simulink model "MCC"  (Simulink 9.0)
settings: Solver=ode15s  StartTime=0.0  StopTime=0.2  RelTol=1e-3
InitFcn:
  | MCC_constants
StartFcn:
  | MCC_constants
values from neighbouring files (symbols this model uses):
  b = 8.5E-3    (= 0.0085)    [TD2_config.m]
  J = 0.28    [TD2_config.m]
  K = 0.5093    [TD2_config.m]
  L = 1.6E-3    (= 0.0016)    [TD2_config.m]
  R = 0.13    [TD2_config.m]
settings Model: Creator=TABLE 6  LastModifiedBy=TABLE 6
settings DataIOCC: SaveFormat=Dataset
settings OptimizationCC: LifeSpan=auto
settings DebuggingCC: UnderspecifiedInitializationDetection=Simplified  MergeDetectMultiDrivingBlocksExec=error  SFUnexpectedBacktrackingDiag=error  SFNoUnconditionalDefaultTransitionDiag=error  SFExecutionAtInitializationDiag=warning
settings HardwareCC: ProdBitPerPointer=64  ProdBitPerSizeT=64  ProdBitPerPtrDiffT=64  ProdLargestAtomicFloat=Float  ProdIntDivRoundTo=Zero  ProdEndianess=LittleEndian  ProdWordSize=64  ProdHWDeviceType=Intel->x86-64 (Windows64)
settings ModelReferenceCC: PropagateSignalLabelsOutOfModel=on
settings CodeAppCC: StateflowObjectComments=off
settings GRTTargetCC: TargetLangStandard=C99 (ISO)
settings ConfigComp: CovMetricSettings=dwe  CovHtmlReporting=off  CovSaveCumulativeToWorkspaceVar=off  CovSaveSingleToWorkspaceVar=off  CovExternalEMLEnable=on

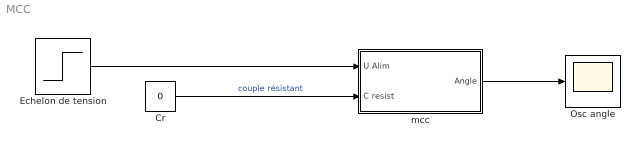
== system MCC ==
  Cr : Constant  Value=0
  Echelon de tension : Step  Time=0  After=12  SampleTime=0
  "Osc angle  " : Scope
  mcc : Subsystem
  wires:
  Echelon de tension/1 -> mcc/1(U Alim)
  Cr/1 -> mcc/2(C resist)  "couple résistant"
  mcc/1(Angle) -> "Osc angle  "/1

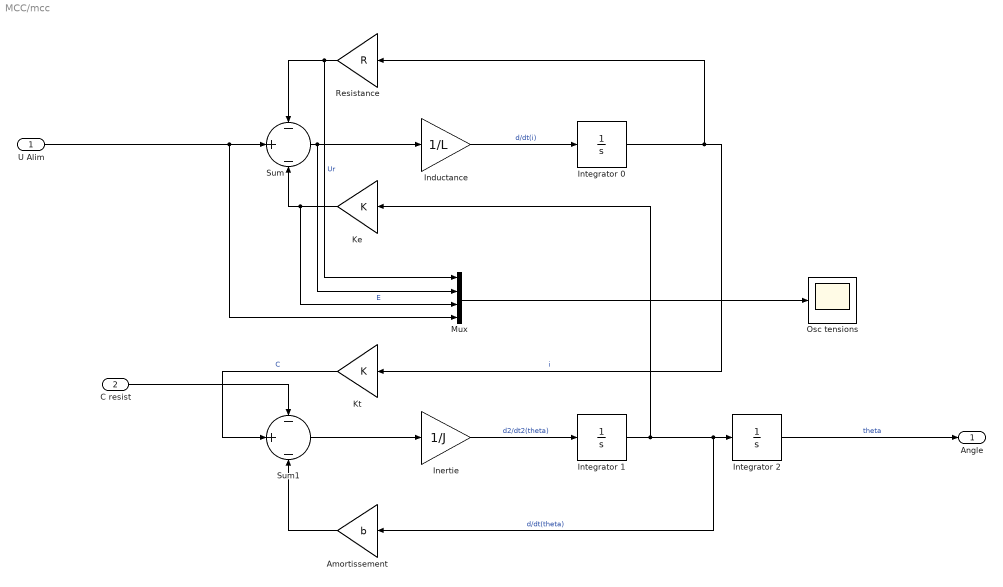
== system MCC/mcc ==
  U Alim : Inport
  C resist : Inport  Port=2
  "\tAmortissement" : Gain  Gain=b
  "\tInductance" : Gain  Gain=1/L
  "\tInertie" : Gain  Gain=1/J
  "\tKe" : Gain  Gain=K
  "\tKt" : Gain  Gain=K
  "\tResistance" : Gain  Gain=R
  Integrator 0 : Integrator
  "Integrator 1 " : Integrator
  "Integrator 2 " : Integrator
  Mux : Mux
  Osc tensions : Scope
  Sum : Sum  Inputs=-|+|-
  Sum1 : Sum  Inputs=-|+|-
  Angle : Outport
  wires:
  "Integrator 2 "/1 -> Angle/1  "theta"
  "\tResistance"/1 -> Mux/1, Sum/1  "Ur"
  C resist/1 -> Sum1/1
  Mux/1 -> Osc tensions/1
  "\tAmortissement"/1 -> Sum1/3
  "\tKe"/1 -> Mux/3, Sum/3  "E"
  "\tKt"/1 -> Sum1/2  "C"
  Integrator 0/1 -> "\tResistance"/1, "\tKt"/1  "i"
  "\tInertie"/1 -> "Integrator 1 "/1  "d2/dt2(theta)"
  Sum1/1 -> "\tInertie"/1
  U Alim/1 -> Mux/4, Sum/2
  "Integrator 1 "/1 -> "\tKe"/1, "\tAmortissement"/1, "Integrator 2 "/1  "d/dt(theta)"
  Sum/1 -> Mux/2, "\tInductance"/1
  "\tInductance"/1 -> Integrator 0/1  "d/dt(i)"
